simulink model "Day2_3_rate_limiter"  (R2022b)
settings: Solver=FixedStepAuto  StartTime=0.0  StopTime=10.0  FixedStep=0.001  RelTol=1e-3
InitFcn:
  | a = 10;
  | Ts = 0.001;
settings Model: Creator=user  LastModifiedBy=user

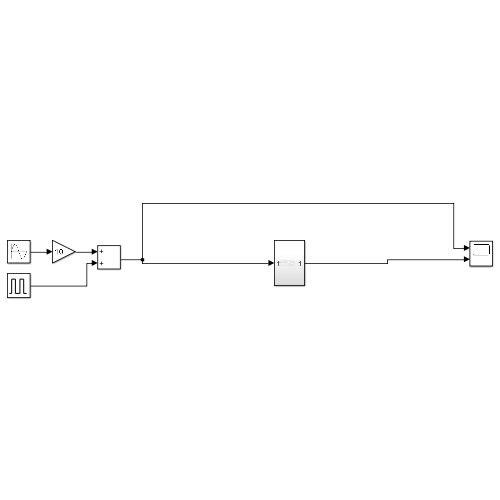
[thumbnail: Simulink's stored preview of the top-level diagram]
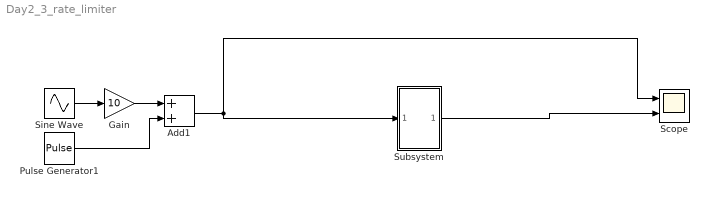
== system Day2_3_rate_limiter ==
  Add1 : Sum
  Gain : Gain  Gain=10
  Pulse Generator1 : DiscretePulseGenerator  PulseType=Time based  Amplitude=5  Period=5  PulseWidth=5  PhaseDelay=1
  Scope : Scope  NumInputPorts=2
  Sine Wave : Sin  SampleTime=0
  Subsystem : Subsystem
  wires:
  Sine Wave/1 -> Gain/1
  Gain/1 -> Add1/1
  Pulse Generator1/1 -> Add1/2
  Add1/1 -> Subsystem/1(In1), Scope/1
  Subsystem/1(Out1) -> Scope/2

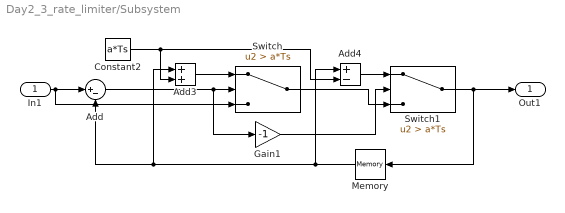
== system Day2_3_rate_limiter/Subsystem ==
  In1 : Inport
  Add : Sum  Inputs=|+-
  Add3 : Sum
  Add4 : Sum  Inputs=+-
  Constant2 : Constant  Value=a*Ts
  Gain1 : Gain  Gain=-1
  Memory : Memory
  Switch : Switch  Criteria=u2 > Threshold  Threshold=a*Ts  SaturateOnIntegerOverflow=off  InputSameDT=off
  Switch1 : Switch  Criteria=u2 > Threshold  Threshold=a*Ts  SaturateOnIntegerOverflow=off  InputSameDT=off
  Out1 : Outport
  wires:
  Switch/1 -> Switch1/3
  Constant2/1 -> Add4/2, Add3/2
  Switch1/1 -> Out1/1, Memory/1
  Memory/1 -> Add/2, Add3/1, Add4/1
  Add4/1 -> Switch1/1
  Gain1/1 -> Switch1/2
  Add3/1 -> Switch/1
  Add/1 -> Switch/2, Gain1/1
  In1/1 -> Add/1, Switch/3
